simulink model "compare_lin_non_lin"  (R2021b)
settings: Solver=FixedStepAuto  StartTime=0.0  StopTime=10  FixedStep=0.001  RelTol=1e-3
values from neighbouring files (symbols this model uses):
  A = [0 0.279152395567 0 -266.21056686 0 1 -102.549528262 0 379.754001356 0 0 0.401529598058 ... (25 elements, 5x5)]    [System.mat]    (also in linearize_operating_point.m = double(A))
  B = [0 0 0 0 5076.90787281]    [System.mat]    (also in linearize_operating_point.m = double(B))
  C = [1  0  0  0  0; 0  0  1  0  0]    [System.mat]    (also in linearize_operating_point.m = [1 0 0 0 0)
  D = [0 0]    [System.mat]    (also in linearize_operating_point.m = zeros(2,1))
  params = [9.81 0.1 0.1 0.125 0.05 -0.0300000121036 0.030345196835 0.100000000002 1.00882387117e-05 10.2757053002 1.78577414601e-05 65.9998023467 ... (13 elements, 1x13)]    [System.mat]    (also in linearize_operating_point.m = [9.81, 0.1, 0.1, 0.125, 0.05, -0.0300000121036330, 0.0303451)
  theta_1_0 = x_op(1)    [controller.m]    (also in run_compare_lin_non_lin.m)
  theta_2_0 = x_op(3)    [controller.m]    (also in run_compare_lin_non_lin.m)
  x_op = [3.14159265359 0 0 0 0]    [System.mat]    (also in linearize_operating_point.m = [init_theta_1; 0; init_theta_2; 0; 0])
settings Model: Creator=annel  LastModifiedBy=lyitingli
settings DebuggingCC: UnconnectedInputMsg=none  UnconnectedOutputMsg=none  UnconnectedLineMsg=none
settings ModelReferenceCC: EnableRefExpFcnMdlSchedulingChecks=off
settings RTWCC: DLArmComputeVersion=20.02.1

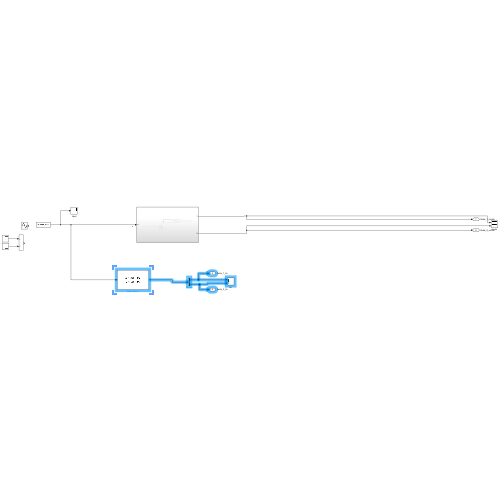
[thumbnail: Simulink's stored preview of the top-level diagram]
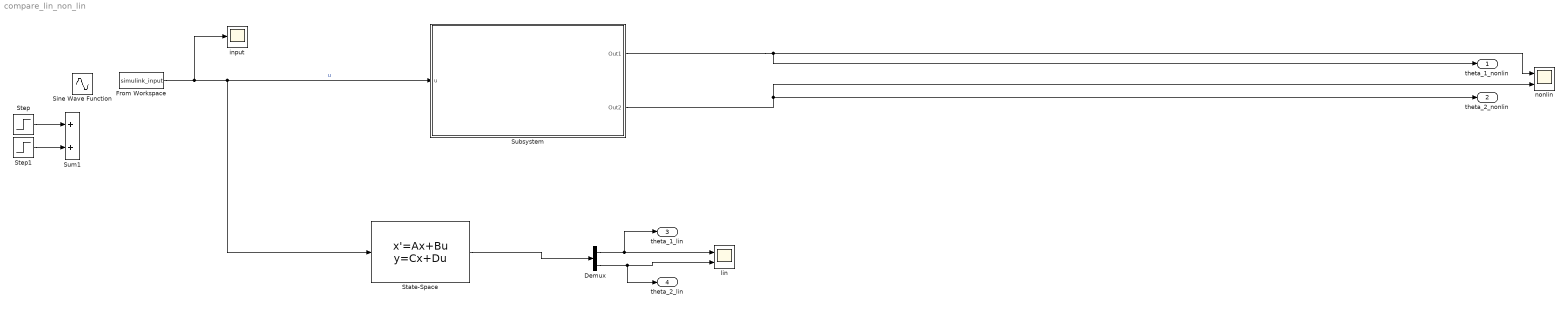
== system compare_lin_non_lin ==
  Demux : Demux  Outputs=2
  From Workspace : FromWorkspace  SampleTime=-1
  Sine Wave Function : Sin  Amplitude=0.05  Frequency=2*pi*2  SampleTime=0.001
  State-Space : StateSpace  A=A  B=B  C=C  D=D  InitialCondition=x_op-x_op
  Step : Step  Time=0
  Step1 : Step  Time=0.05  After=-1
  Subsystem : Subsystem
  Sum1 : Sum
  input : Scope
  lin : Scope  NumInputPorts=2
  nonlin : Scope  NumInputPorts=2
  theta_1_nonlin : Outport
  theta_2_nonlin : Outport  Port=2
  theta_1_lin : Outport  Port=3
  theta_2_lin : Outport  Port=4
  wires:
  Demux/1 -> theta_1_lin/1, lin/1
  Demux/2 -> lin/2, theta_2_lin/1
  State-Space/1 -> Demux/1
  Step1/1 -> Sum1/2
  Step/1 -> Sum1/1
  From Workspace/1 -> State-Space/1, Subsystem/1(u), input/1  "u"
  Subsystem/1(Out1) -> theta_1_nonlin/1, nonlin/1
  Subsystem/2(Out2) -> nonlin/2, theta_2_nonlin/1

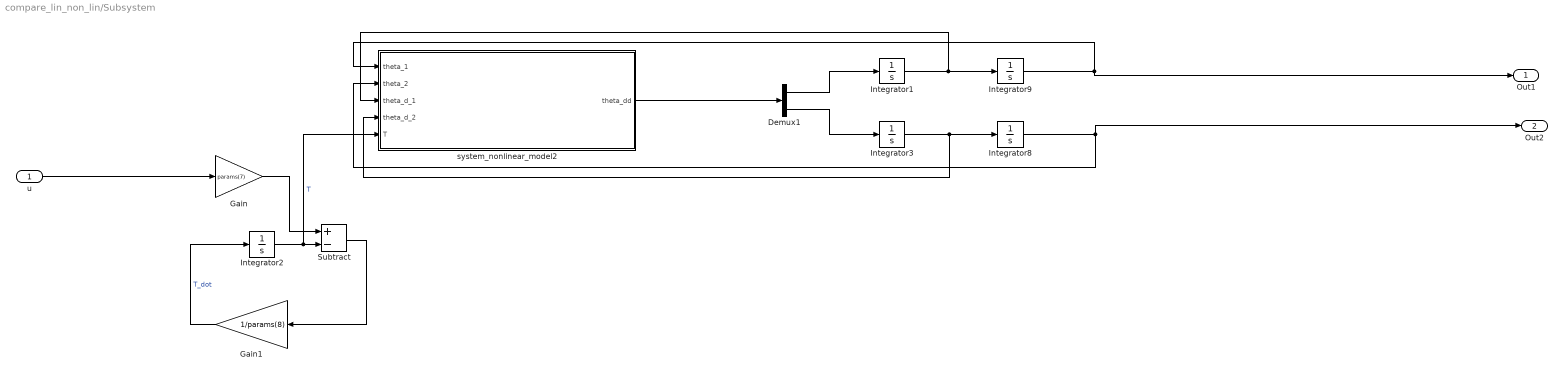
== system compare_lin_non_lin/Subsystem ==
  u : Inport
  Demux1 : Demux  Outputs=2
  Gain : Gain  Gain=params(7)
  Gain1 : Gain  Gain=1/params(8)
  Integrator1 : Integrator
  Integrator2 : Integrator
  Integrator3 : Integrator
  Integrator8 : Integrator  InitialCondition=theta_2_0
  Integrator9 : Integrator  InitialCondition=theta_1_0
  Subtract : Sum  Inputs=+-
  system_nonlinear_model2 : MATLAB Function  TreatAsAtomicUnit=on
  Out1 : Outport
  Out2 : Outport  Port=2
  wires:
  Demux1/2 -> Integrator3/1
  Integrator1/1 -> system_nonlinear_model2/3(theta_d_1), Integrator9/1
  Integrator3/1 -> system_nonlinear_model2/4(theta_d_2), Integrator8/1
  system_nonlinear_model2/1(theta_dd) -> Demux1/1
  Integrator9/1 -> Out1/1, system_nonlinear_model2/1(theta_1)
  Integrator8/1 -> Out2/1, system_nonlinear_model2/2(theta_2)
  Subtract/1 -> Gain1/1
  Demux1/1 -> Integrator1/1
  Gain1/1 -> Integrator2/1  "T_dot"
  Gain/1 -> Subtract/1
  Integrator2/1 -> system_nonlinear_model2/5(T), Subtract/2  "T"
  u/1 -> Gain/1

== matlab function compare_lin_non_lin/Subsystem/system_nonlinear_model2 ==
  settings: updateMethod=DISCRETE  sampleTime=0.001
  data: theta_dd output size=2; theta_1 input size=1; theta_2 input size=1; theta_d_1 input size=1; theta_d_2 input size=1; T input size=1
function theta_dd    = get_theta_dt_dt(theta_1, theta_2, theta_d_1, theta_d_2, T)


% constant variables
g = 9.81;
l_1 = 0.1;
l_2 = 0.1;
m_1 = 0.125;
m_2 = 0.05;
% params = [-0.04, 0.06, 0.074, 0.00002, 4.8, 0.00077, 50, 0.03];
params = [0 -0.0300000121036330, 0.0303451968350115, 0.1000000000017210, 1.00882387117299e-05, 10.27570530021582, 1.78577414601457e-05, 65.9998023466922, 0.01300000000002200];


% varying variables

c_1_0 = params(2);
c_2_0 = params(3);
I_1_0 = params(4);
I_2_0 = params(5);
b_1_0 = params(6);
b_2_0 = params(7);
k_m_0 = params(8);
tau_e_0 = params(9);


theta_dd = [                                                                                                                                                                                                               theta_d_2*((200*b_2_0*(10*c_2_0^2 + cos(theta_2)*c_2_0 + 200*I_2_0))/(20*I_2_0 - c_2_0^2*cos(theta_2)^2 + 2000*I_1_0*c_2_0^2 + 5000*I_2_0*c_1_0^2 + c_2_0^2 + 250*c_1_0^2*c_2_0^2 + 40000*I_1_0*I_2_0) + (10*c_2_0*sin(theta_2)*(theta_d_1 + theta_d_2)*(c_2_0^2 + 20*I_2_0))/(20*I_2_0 - c_2_0^2*cos(theta_2)^2 + 2000*I_1_0*c_2_0^2 + 5000*I_2_0*c_1_0^2 + c_2_0^2 + 250*c_1_0^2*c_2_0^2 + 40000*I_1_0*I_2_0)) - theta_d_1*((2000*(c_2_0^2 + 20*I_2_0)*(b_1_0 - (c_2_0*theta_d_2*sin(theta_2))/200))/(20*I_2_0 - c_2_0^2*cos(theta_2)^2 + 2000*I_1_0*c_2_0^2 + 5000*I_2_0*c_1_0^2 + c_2_0^2 + 250*c_1_0^2*c_2_0^2 + 40000*I_1_0*I_2_0) - (c_2_0*theta_d_1*sin(theta_2)*(10*c_2_0^2 + cos(theta_2)*c_2_0 + 200*I_2_0))/(20*I_2_0 - c_2_0^2*cos(theta_2)^2 + 2000*I_1_0*c_2_0^2 + 5000*I_2_0*c_1_0^2 + c_2_0^2 + 250*c_1_0^2*c_2_0^2 + 40000*I_1_0*I_2_0)) + (2000*(sin(theta_1)*((981*c_1_0)/800 + 981/20000) + (981*c_2_0*sin(theta_1 + theta_2))/2000)*(c_2_0^2 + 20*I_2_0))/(20*I_2_0 - c_2_0^2*cos(theta_2)^2 + 2000*I_1_0*c_2_0^2 + 5000*I_2_0*c_1_0^2 + c_2_0^2 + 250*c_1_0^2*c_2_0^2 + 40000*I_1_0*I_2_0) + (2000*T*(c_2_0^2 + 20*I_2_0))/(20*I_2_0 - c_2_0^2*cos(theta_2)^2 + 2000*I_1_0*c_2_0^2 + 5000*I_2_0*c_1_0^2 + c_2_0^2 + 250*c_1_0^2*c_2_0^2 + 40000*I_1_0*I_2_0) - (981*c_2_0*sin(theta_1 + theta_2)*(10*c_2_0^2 + cos(theta_2)*c_2_0 + 200*I_2_0))/(10*(20*I_2_0 - c_2_0^2*cos(theta_2)^2 + 2000*I_1_0*c_2_0^2 + 5000*I_2_0*c_1_0^2 + c_2_0^2 + 250*c_1_0^2*c_2_0^2 + 40000*I_1_0*I_2_0))
theta_d_1*((200*(b_1_0 - (c_2_0*theta_d_2*sin(theta_2))/200)*(10*c_2_0^2 + cos(theta_2)*c_2_0 + 200*I_2_0))/(20*I_2_0 - c_2_0^2*cos(theta_2)^2 + 2000*I_1_0*c_2_0^2 + 5000*I_2_0*c_1_0^2 + c_2_0^2 + 250*c_1_0^2*c_2_0^2 + 40000*I_1_0*I_2_0) - (c_2_0*theta_d_1*sin(theta_2)*(250*c_1_0^2 + 100*c_2_0^2 + 20*cos(theta_2)*c_2_0 + 2000*I_1_0 + 2000*I_2_0 + 1))/(10*(20*I_2_0 - c_2_0^2*cos(theta_2)^2 + 2000*I_1_0*c_2_0^2 + 5000*I_2_0*c_1_0^2 + c_2_0^2 + 250*c_1_0^2*c_2_0^2 + 40000*I_1_0*I_2_0))) - theta_d_2*((20*b_2_0*(250*c_1_0^2 + 100*c_2_0^2 + 20*cos(theta_2)*c_2_0 + 2000*I_1_0 + 2000*I_2_0 + 1))/(20*I_2_0 - c_2_0^2*cos(theta_2)^2 + 2000*I_1_0*c_2_0^2 + 5000*I_2_0*c_1_0^2 + c_2_0^2 + 250*c_1_0^2*c_2_0^2 + 40000*I_1_0*I_2_0) + (c_2_0*sin(theta_2)*(theta_d_1 + theta_d_2)*(10*c_2_0^2 + cos(theta_2)*c_2_0 + 200*I_2_0))/(20*I_2_0 - c_2_0^2*cos(theta_2)^2 + 2000*I_1_0*c_2_0^2 + 5000*I_2_0*c_1_0^2 + c_2_0^2 + 250*c_1_0^2*c_2_0^2 + 40000*I_1_0*I_2_0)) - (200*(sin(theta_1)*((981*c_1_0)/800 + 981/20000) + (981*c_2_0*sin(theta_1 + theta_2))/2000)*(10*c_2_0^2 + cos(theta_2)*c_2_0 + 200*I_2_0))/(20*I_2_0 - c_2_0^2*cos(theta_2)^2 + 2000*I_1_0*c_2_0^2 + 5000*I_2_0*c_1_0^2 + c_2_0^2 + 250*c_1_0^2*c_2_0^2 + 40000*I_1_0*I_2_0) - (200*T*(10*c_2_0^2 + cos(theta_2)*c_2_0 + 200*I_2_0))/(20*I_2_0 - c_2_0^2*cos(theta_2)^2 + 2000*I_1_0*c_2_0^2 + 5000*I_2_0*c_1_0^2 + c_2_0^2 + 250*c_1_0^2*c_2_0^2 + 40000*I_1_0*I_2_0) + (981*c_2_0*sin(theta_1 + theta_2)*(250*c_1_0^2 + 100*c_2_0^2 + 20*cos(theta_2)*c_2_0 + 2000*I_1_0 + 2000*I_2_0 + 1))/(100*(20*I_2_0 - c_2_0^2*cos(theta_2)^2 + 2000*I_1_0*c_2_0^2 + 5000*I_2_0*c_1_0^2 + c_2_0^2 + 250*c_1_0^2*c_2_0^2 + 40000*I_1_0*I_2_0))
 ];
